simulink model "exam2"  (Simulink 7.5)
settings: Solver=ode45  StartTime=0.0  StopTime=20e-3  RelTol=1e-3
undefined symbols (not defined in the file or in its folder): f
libraries: powerlib x9, simulink x2
settings Model: Creator=Sambhav  LastModifiedBy=Sambhav

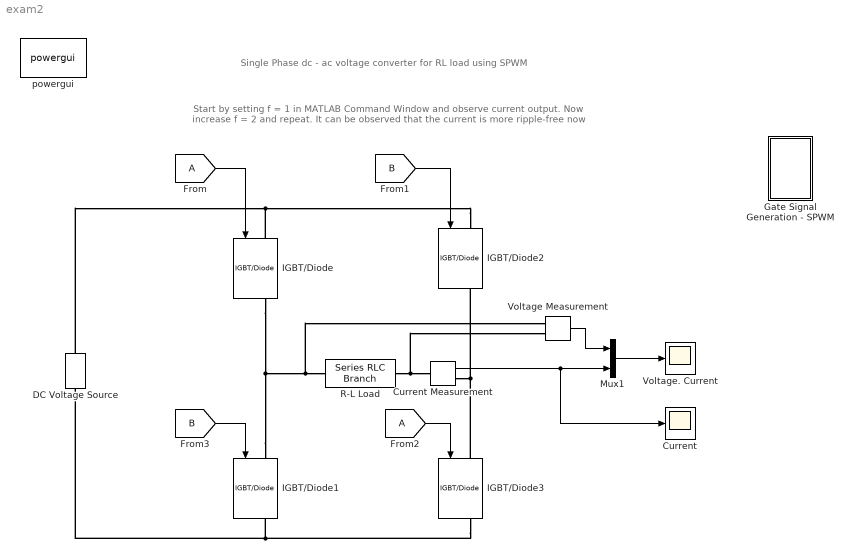
== system exam2 ==
  note: Single Phase dc - ac voltage converter for RL load using SPWM
  note: Start by setting f = 1 in MATLAB Command Window and observe current output.
      | Now increase f = 2 and repeat. It can be observed that the current is more ripple-free now
  Current : Scope
      settings: YMin=-10  YMax=10  SampleInput=on  SampleTime=1e-6
  Current Measurement : powerlib/Measurements/Current Measurement  DialogController=POWERSYS.PowerSysDialog  SystemSampleTime=-1  PhasorSimulation=off  OutputType=Complex  PSBequivalent=0
  DC Voltage Source : powerlib/Electrical Sources/DC Voltage Source  DialogController=POWERSYS.PowerSysDialog  SystemSampleTime=-1  Amplitude=230*sqrt(2)  Measurements=None
  Gate Signal Generation - SPWM : Subsystem
  IGBT/Diode{,1..3} (4 alike) : powerlib/Power Electronics/IGBT//Diode  DialogController=POWERSYS.PowerSysDialog  SystemSampleTime=-1  Ron=1e-3  Rs=1e5  Cs=inf  Measurements=on
  Mux1 : Mux  Inputs=2
  R-L Load : powerlib/Elements/Series RLC Branch  DialogController=POWERSYS.PowerSysDialog  PhysicalDomain=powersysdomain  SubClassName=unknown  LeftPortType=p1  RightPortType=p1  LConnTagsString=__new0  RConnTagsString=__new0  BranchType=RL  Resistance=1  Inductance=1e-3  SetiL0=off  InitialCurrent=0  Capacitance=0  Setx0=off  InitialVoltage=0  Measurements=None
  Voltage Measurement : powerlib/Measurements/Voltage Measurement  DialogController=POWERSYS.PowerSysDialog  SystemSampleTime=-1  PhasorSimulation=off  OutputType=Complex  PSBequivalent=0
  Voltage. Current : Scope
      settings: YMin=-350  YMax=350  SaveName=ScopeData5  SampleInput=on  SampleTime=1e-6
  powergui : powerlib/powergui  Priority=1  SystemSampleTime=-1  SimulationMode=Continuous  SampleTime=50e-6  frequency=60  SPID=off  DisableSnubberDevices=off  DisableRonSwitches=off  DisableVfSwitches=off  SwTol=0  Interpol=off  frequencyindice=0  echomessages=off  HookPort=off  DisplayEquations=off  FunctionMessages=off  EnableUseOfTLC=off  x0status=blocks  RestoreLinks=warning  ResistiveCurrentMeasurement=off  Ylog=off  Xlog=on  ShowGrid=off  save=off  variable=ZData  ZoomFFT=off  StartTime=0.0  cycles=1  DisplayStyle=1  FreqAxis=off  MaxFrequency=1000  frequencyindicesteady=1  display=off  methode=off
  wires:
  [B] -> IGBT/Diode2/1
  [A] -> IGBT/Diode/1
  [A] -> IGBT/Diode3/1
  Mux1/1 -> Voltage. Current/1
  Voltage Measurement/1 -> Mux1/1
  Current Measurement/1 -> Mux1/2, Current/1
  [B] -> IGBT/Diode1/1
  connections:
  IGBT/Diode1/LConn1 -- R-L Load/LConn1 -- Voltage Measurement/LConn1 -- IGBT/Diode/RConn1
  IGBT/Diode2/LConn1 -- DC Voltage Source/RConn1 -- IGBT/Diode/LConn1
  IGBT/Diode3/RConn1 -- DC Voltage Source/LConn1 -- IGBT/Diode1/RConn1
  IGBT/Diode3/LConn1 -- Current Measurement/RConn1 -- IGBT/Diode2/RConn1
  R-L Load/RConn1 -- Current Measurement/LConn1 -- Voltage Measurement/LConn2

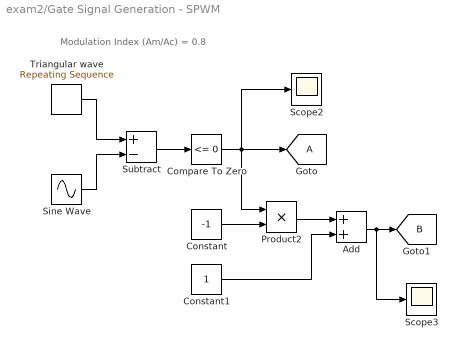
== system exam2/Gate Signal Generation - SPWM ==
  note: Modulation Index (Am/Ac) = 0.8
  Add : Sum  OutDataType=fixdt(1, 16)  OutScaling=2^-10
  Compare To Zero : simulink/Logic and Bit Operations/Compare To Zero  SystemSampleTime=-1  relop=<=  LogicOutDataTypeMode=uint8
  Constant : Constant  Value=-1  OutDataType=fixdt(1, 16)  OutScaling=2^0
  Constant1 : Constant  OutDataType=fixdt(1, 16)  OutScaling=2^0
  Product2 : Product  OutDataType=fixdt(1, 16)  OutScaling=2^0  RndMeth=Zero
  Scope2 : Scope
      settings: SaveName=ScopeData2  SampleInput=on  SampleTime=1e-6
  Scope3 : Scope
      settings: SaveName=ScopeData3  SampleInput=on  SampleTime=1e-6
  Sine Wave : Sin  Amplitude=8  Bias=0  Frequency=100*pi  Phase=0  Samples=10  SampleTime=0  Offset=0
  Subtract : Sum  Inputs=+-  OutDataType=fixdt(1, 16)  OutScaling=2^-10
  Triangular wave : simulink/Sources/Repeating Sequence  SystemSampleTime=-1  rep_seq_t=[0 0.25e-3/f 0.75e-3/f 1e-3/f]  rep_seq_y=[0 10 -10 0]
  tag scope: A=global, B=global
  wires:
  Subtract/1 -> Compare To Zero/1
  Triangular wave/1 -> Subtract/1
  Sine Wave/1 -> Subtract/2
  Compare To Zero/1 -> Product2/1, [A], Scope2/1
  Constant/1 -> Product2/2
  Product2/1 -> Add/1
  Constant1/1 -> Add/2
  Add/1 -> [B], Scope3/1
